simulink model "clean"  (R2016b)
settings: Solver=VariableStepAuto  StartTime=0.0  StopTime=200  RelTol=1e-3
libraries: simulink x2
settings Model: Creator=kefin  LastModifiedBy=kefin

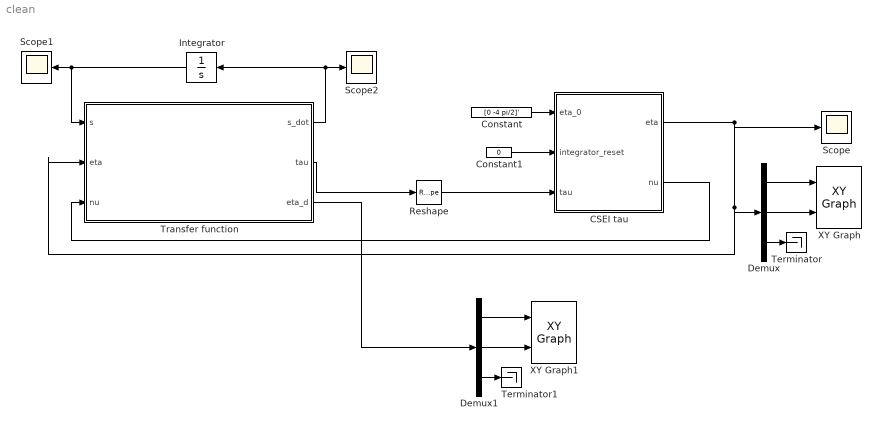
== system clean ==
  CSEI tau : Subsystem
  Constant : Constant  Value=[0 -4 pi/2]'
  Constant1 : Constant  Value=0
  Demux : Demux  Outputs=3
  Demux1 : Demux  Outputs=3
  Integrator : Integrator  UpperSaturationLimit=1  LowerSaturationLimit=0
  Reshape : Reshape  OutputDimensionality=Customize  OutputDimensions=[3,1]
  Scope : Scope
  Scope1 : Scope
  Scope2 : Scope
  Terminator : Terminator
  Terminator1 : Terminator
  Transfer function : MATLAB Function  TreatAsAtomicUnit=on
  XY Graph : simulink/Sinks/XY Graph  xmin=-20  xmax=20  ymin=-20  ymax=20  st=-1
  XY Graph1 : simulink/Sinks/XY Graph  xmin=-20  xmax=20  ymin=-20  ymax=20  st=-1
  wires:
  Transfer function/1(s_dot) -> Integrator/1, Scope2/1
  Integrator/1 -> Scope1/1, Transfer function/1(s)
  Constant/1 -> CSEI tau/1(eta_0)
  Constant1/1 -> CSEI tau/2(integrator_reset)
  Transfer function/2(tau) -> Reshape/1
  CSEI tau/2(nu) -> Transfer function/3(nu)
  CSEI tau/1(eta) -> Transfer function/2(eta), Demux/1, Scope/1
  Reshape/1 -> CSEI tau/3(tau)
  Demux/1 -> XY Graph/1
  Demux/2 -> XY Graph/2
  Demux/3 -> Terminator/1
  Transfer function/3(eta_d) -> Demux1/1
  Demux1/1 -> XY Graph1/1
  Demux1/2 -> XY Graph1/2
  Demux1/3 -> Terminator1/1

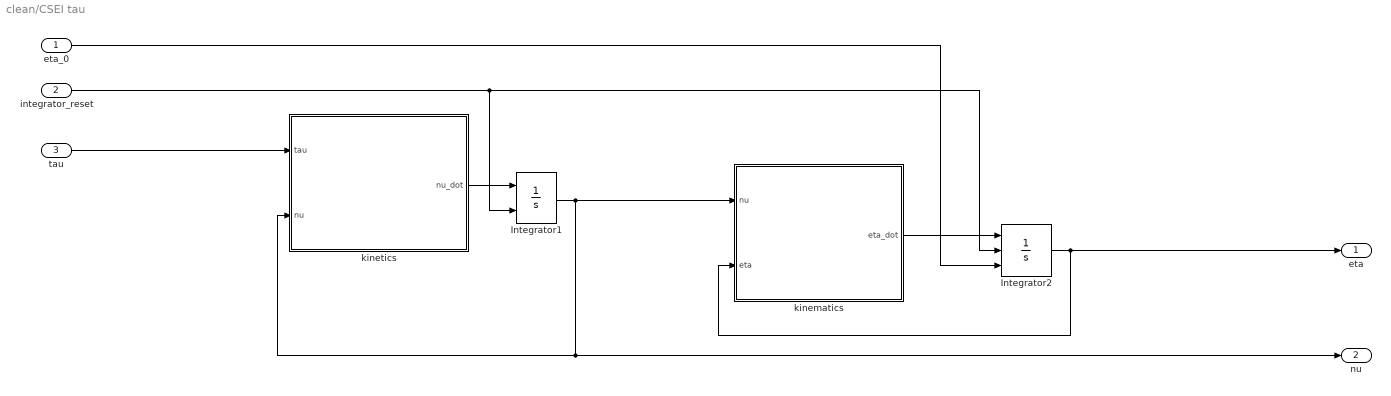
== system clean/CSEI tau ==
  eta_0 : Inport
  integrator_reset : Inport  Port=2
  tau : Inport  Port=3
  Integrator1 : Integrator  ExternalReset=rising  InitialCondition=[0 0 0]'
  Integrator2 : Integrator  ExternalReset=rising  InitialConditionSource=external  InitialCondition=[0 0 0]'
  kinematics : MATLAB Function  TreatAsAtomicUnit=on
  kinetics : MATLAB Function  TreatAsAtomicUnit=on
  eta : Outport
  nu : Outport  Port=2
  wires:
  Integrator1/1 -> nu/1, kinetics/2(nu), kinematics/1(nu)
  tau/1 -> kinetics/1(tau)
  kinetics/1(nu_dot) -> Integrator1/1
  integrator_reset/1 -> Integrator2/2, Integrator1/2
  Integrator2/1 -> eta/1, kinematics/2(eta)
  eta_0/1 -> Integrator2/3
  kinematics/1(eta_dot) -> Integrator2/1

== matlab function clean/CSEI tau/kinematics ==
  data: nu input; eta_dot output; eta input
function eta_dot = CSE1_eta_dot(nu,eta)

psi = eta(3);

J = [cos(psi) -sin(psi) 0
     sin(psi) cos(psi)  0
     0        0         1];

eta_dot = J*nu;

== matlab function clean/Transfer function ==
  data: s input; eta input; nu input; s_dot output; tau output; eta_d output
function [s_dot, tau, eta_d] = maneuver(s, eta, nu)
%% Constants
P_d = [2 0; 10 4];
mu = 0.1;
K_p = diag([0.2 0.2 0.1]);
K_2 = 10*eye(3); K_2(3, 3) = K_2(3, 3) / 2;
U_max = 4;

%% Parameters
% Rigid body and added mass
m = 14.79; 
I_z = 1.76; 
x_g = 0.0375; 
% y_g = 0.0;

X_u_dot = -2; 
Y_v_dot = -10; 
Y_r_dot = -0; 
N_r_dot = -1; 

% Max Values in Surge X, Sway Y and Yaw N
X_max = 1.03; %[N]
Y_max = 0.98; %[N]
N_max = 2.50; %[Nm]


% Hydro surge, Hydro sway and Hydro Yaw Parameters
    % NB! We don't need most of them for now, that why they are commented
    % out, but don't remove them!!
X_u = -0.6555;  Y_v = -1.33;    N_v = 0.0; 
X_uu = 0.3545;  Y_vv = -2.776;  N_vv = -0.2088; 
X_uuu = -3.787; Y_vvv = -64.91; N_vvv = 0.0;
X_v = 0.0;      Y_r = -7.25;    N_r = -1.9; 
X_vv = -2.443;  Y_rr = -3.45;   N_rr = 0.75;
X_vvv = 0.0;    Y_rrr = 0.0;    N_rrr = 0.0;
                Y_rv = 0.805;   N_rv = 0.130;
                Y_vr = -0.845;  N_vr = 0.080;
      
% Matrices
u = nu(1); v = nu(2); r = nu(3); % I need a test values; 
    
a_11 = m-X_u_dot;   a_12 = 0;                   a_13 = 0; 
a_21 = 0;           a_22 = m-Y_v_dot ;          a_23 = m*x_g - Y_r_dot;
a_31 = 0;           a_32 = m*x_g - Y_r_dot;     a_33 = I_z - N_r_dot;

M = [a_11 a_12, a_13; a_12 a_22 a_23; a_31 a_32 a_33];

d_11_u =  -X_u - X_uu*abs(u) - X_uuu*u^2;
d_22_vr = -Y_v - Y_vv*abs(v) - Y_vvv*v^2   - Y_rv*abs(r);
d_23_vr = -Y_r - Y_vr*abs(v) - Y_rr*abs(r) - Y_rrr*r^2;
d_32_vr = -N_v - N_vv*abs(v) - N_vvv*v^2   - N_rv*abs(r);
d_33_vr = -N_r - N_vr*abs(v) - N_rr*abs(r) - N_rrr*r^2;

% The total damping matrix from the handbook page 53
D_tot = [d_11_u 0 0; 0 d_22_vr d_23_vr; 0 d_32_vr d_33_vr];

switch 4
    case 1
        %% Straight line
        %% Speed mapping
        U_ref = U_max / 5;
        U_s = U_ref / sqrt(sum((P_d(:,2)-P_d(:,1)).^2));
        U_s_s = 0;

        %% Reference mapping
        p_d = max(min(s,1),0).*[P_d(2,1) - P_d(1,1); P_d(2,2) - P_d(1,2)] + [P_d(1,1); P_d(1,2)];
        psi_d = atan2(P_d(2,2) - P_d(1,2), P_d(2,1) - P_d(1,1));

        p_d_s = [P_d(2,1) - P_d(1,1); P_d(2,2) - P_d(1,2)];
        psi_d_s = 0;

        p_d_ss = [0; 0];
        psi_d_ss = 0;

        eta_d = [p_d; psi_d];
        eta_d_s = [p_d_s; psi_d_s];
        eta_d_ss = [p_d_ss; psi_d_ss];

        %% Update law
        diff = eta - eta_d; diff(3) = angdiff(eta_d(3), eta(3));
        if norm(eta_d_s) < 1e-5
            s_dot = U_s - mu * -diff' * ones(3,1) / norm(ones(3, 1));
        else
            s_dot = U_s - mu * -diff' * eta_d_s / norm(eta_d_s);
        end
        if s >= 1
            s_dot = 0;
            eta_d_s = eta_d_s*0;
        end
    case 2
        %% Forward and backward on a straight line
        %% Speed mapping
        U_ref = U_max / 5;
        U_s = U_ref / sqrt(sum((P_d(:,2)-P_d(:,1)).^2));
        U_s_s = 0;

        %% Reference mapping
        % These work, but go out of bounds below.
        multiplicant    = sin(s);
        derivicant      = cos(s);
        superderivicant = -sin(s);
        
        p_d = multiplicant*[P_d(2,1) - P_d(1,1); P_d(2,2) - P_d(1,2)]/2 + [P_d(2,1) - P_d(1,1); P_d(2,2) - P_d(1,2)]/2;
        psi_d = atan2(P_d(2,2) - P_d(1,2), P_d(2,1) - P_d(1,1));

        p_d_s = derivicant*[(P_d(2,1) - P_d(1,1)); (P_d(2,2) - P_d(1,2))]/2;
        psi_d_s = 0;

        p_d_ss = superderivicant*[(P_d(2,1) - P_d(1,1)); (P_d(2,2) - P_d(1,2))]/2;
        psi_d_ss = 0;

        eta_d = [p_d; psi_d];
        eta_d_s = [p_d_s; psi_d_s];
        eta_d_ss = [p_d_ss; psi_d_ss];

        %% Update law
        diff = eta - eta_d; diff(3) = angdiff(eta_d(3), eta(3));
        if norm(eta_d_s) < 1e-5
            s_dot = U_s - mu * -diff' * ones(3,1) / norm(ones(3, 1));
        else
            s_dot = U_s - mu * -diff' * eta_d_s / norm(eta_d_s);
        end
    case 3
        %% Forward and backward on a straight line with sinusoidal parametrization of U_ref
        %% Speed mapping
        U_ref = U_max / 5 * (1.01 + sin(2*pi*s - pi/2));
        U_s = U_ref / sqrt(sum((P_d(:,2)-P_d(:,1)).^2));
        U_s_s = 0;

        %% Reference mapping
        multiplicant    = sin(s);
        derivicant      = cos(s);
        superderivicant = -sin(s);
        
        p_d = multiplicant*[P_d(2,1) - P_d(1,1); P_d(2,2) - P_d(1,2)]/2 + [P_d(2,1) - P_d(1,1); P_d(2,2) - P_d(1,2)]/2;
        psi_d = atan2(P_d(2,2) - P_d(1,2), P_d(2,1) - P_d(1,1));

        p_d_s = derivicant*[(P_d(2,1) - P_d(1,1)); (P_d(2,2) - P_d(1,2))]/2;
        psi_d_s = 0;

        p_d_ss = superderivicant*[(P_d(2,1) - P_d(1,1)); (P_d(2,2) - P_d(1,2))]/2;
        psi_d_ss = 0;

        eta_d = [p_d; psi_d];
        eta_d_s = [p_d_s; psi_d_s];
        eta_d_ss = [p_d_ss; psi_d_ss];

        %% Update law
        diff = eta - eta_d; diff(3) = angdiff(eta_d(3), eta(3));
        if norm(eta_d_s) < 1e-5
            s_dot = U_s - mu * -diff' * ones(3,1) / norm(ones(3, 1));
        else
            s_dot = U_s - mu * -diff' * eta_d_s / norm(eta_d_s);
        end
    case 4
        %% Ellipse tracking
        C = [5; 0];
        
        %% Speed mapping
        rx = 5;
        ry = 3;
        U_ref = U_max / 10;
        U_s = U_ref / sqrt((rx*sin(s))^2 + (ry*cos(s))^2);
        U_s_s = -(rx^2*cos(s)*sin(s) - ry^2*cos(s)*sin(s))*U_ref/(ry^2*cos(s)^2 + rx^2*sin(s)^2)^(3/2);

        %% Reference mapping
        p_d = [rx*cos(s)+C(1); ry*sin(s)+C(2)];
        psi_d = atan2(ry*cos(s), -rx*sin(s));

        p_d_s = [-rx*sin(s); ry*cos(s)];
        psi_d_s = rx*ry/(ry^2*cos(s)^2+rx^2*sin(s)^2);

        p_d_ss = [-rx*cos(s); -ry*sin(s)];
        psi_d_ss = -2*(rx^2*cos(s)*sin(s) - ry^2*cos(s)*sin(s))*rx*ry/(ry^2*cos(s)^2 + rx^2*sin(s)^2)^2;

        eta_d = [p_d; psi_d];
        eta_d_s = [p_d_s; psi_d_s];
        eta_d_ss = [p_d_ss; psi_d_ss];

        %% Update law
        diff = eta - eta_d; diff(3) = angdiff(eta_d(3), eta(3));
        if norm(eta_d_s) < 1e-5
            s_dot = U_s - mu * -diff' * ones(3,1) / norm(ones(3, 1));
        else
            s_dot = U_s - mu * -diff' * eta_d_s / norm(eta_d_s);
        end
    otherwise
        disp('Invalid case');
end


%% Control law
% Define z_1 and z_1_dot
S = [0 -r 0; r 0 0; 0 0 0];
psi = eta(3);
R = [cos(psi) -sin(psi) 0;
     sin(psi) cos(psi)  0;
     0        0         1];
 
z_1_a = eta - eta_d;
z_1_psi = angdiff(eta_d(3), eta(3));
z_1_a(3) = z_1_psi;
z_1 = R'*z_1_a;
z_1_dot = S'*z_1 + nu - R'*eta_d_s*s_dot;

% alpha_1, alpha_1_dot, and z_2
alpha_1 = -K_p*z_1 + R'*eta_d_s*U_s;
z_2 = nu - alpha_1;
alpha_1_dot = -K_p*z_1_dot + S'*R'*eta_d_s*U_s + R'*eta_d_ss*s_dot*U_s + R'*eta_d_s*U_s_s*s_dot;

tau = D_tot*nu + M*alpha_1_dot - z_1 - K_2*z_2;
tau = min([X_max Y_max N_max]', tau);
tau = max(-[X_max Y_max N_max]', tau);

function diff = angdiff(alpha, beta)
diff = mod(beta - alpha + pi, 2*pi) - pi;

== matlab function clean/CSEI tau/kinetics ==
  data: tau input; nu_dot output; nu input
function nu_dot = CSE1_nu_dot(tau,nu)

u   = nu(1);
v   = nu(2);
r   = nu(3);

tau = [tau(1);tau(2);tau(3)];
%% MATRICES

m    = 14.79;   I_z  =  1.7600;   x_g = 0.0375;       % x_g  =  0.0460; % Table B.1


%% Added mass
X_ud  =     -2.0;											% Table B.1
					Y_vd =     -1.0;	N_vd =    -0.0;		% Table B.1 guestimate
					Y_rd =      -0.0;	N_rd =    -1.0;		% Table B.1

%% Total mass matrix
m_11 = m-X_ud;
m_22 = m-Y_vd;
m_23 = m*x_g-Y_rd;
m_32 = m*x_g-N_vd;
m_33 = I_z-N_rd;

M    = [m_11 0    0
        0    m_22 m_23
        0    m_32 m_33];
	
%% Damping coefficients
% Comments at the end of the lines indicate the old values used.
X_u		= -0.6555;		X_v		= 0;
X_uu 	= 0.3545;		X_vv	= -2.443;
X_uuu 	= -3.787;		X_vvv	= 0;

						Y_v		= -1.33; 			Y_r		= -7.250; % Y_r
						Y_vv	= -2.776;			Y_rr	= -3.450; % Y_rr
						Y_vvv	= -64.91;			Y_rrr	= 0;
						
						Y_rv	= -0.805;			Y_vr	= -0.845; % Y_rv, Y_vr

						N_v		= 0;				N_r		= -1.900; % N_r
						N_vv	= -0.2088;			N_rr	= -0.750; % N_rr
						N_vvv	= 0;				N_rrr	= 0;
						
						N_rv	= 0.130;			N_vr	= 0.080; % N_rv, N_vr

%% Correolis matrix
c_13 = -(m-Y_vd)*v-(m*x_g-Y_rd)*r;
c_23 = (m-X_ud)*u;
C    = [0     0     c_13
        0     0     c_23
        -c_13 -c_23 0   ];

%% Assembly of the damping matrix
d_11 = -X_u - X_uu*u - X_uuu*u^2;
d_22 = -Y_v - Y_vv*v - Y_vvv*v^2 - Y_rv*abs(r);
d_33 = -N_r - N_rr*abs(r) - N_rrr*r^2 - N_vr*abs(v); % using abs(r)

d_12 = -X_v - X_vv*v - X_vvv*v^2;
d_23 = -Y_r - Y_rr*abs(r) - Y_rrr*r^2 - Y_vr*abs(v);
d_32 = -N_v - N_vv*v - N_vvv*v^2 - N_rv*abs(r);

D    = [d_11 d_12 0
        0    d_22 d_23
        0    d_32 d_33];



%% CALCULATION
nu_dot = M\(tau-(C+D)*nu);
